simulink model "untitled"  (Simulink 7.3)
settings: Solver=ode45  StartTime=0.0  StopTime=10.0  RelTol=1e-3
settings Model: Creator=Sain  LastModifiedBy=Sain

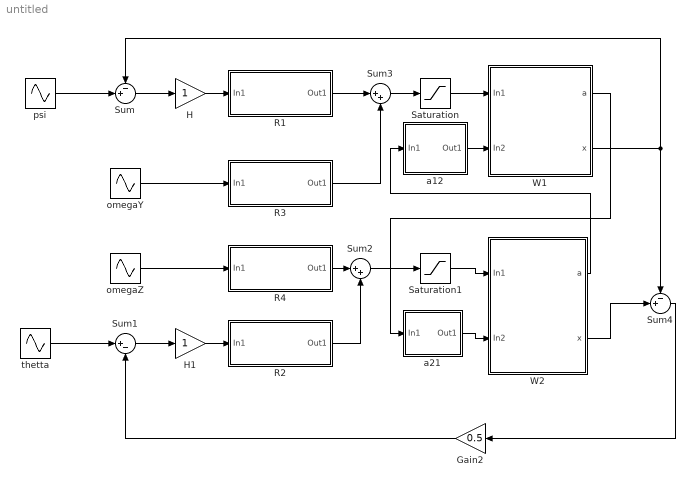
== system untitled ==
  Gain2 : Gain  Gain=0.5  ParameterDataType=fixdt(1, 16)  ParameterScaling=2^0  OutDataType=fixdt(1, 16)  OutScaling=2^0
  H : Gain  ParameterDataType=fixdt(1, 16)  ParameterScaling=2^0  OutDataType=fixdt(1, 16)  OutScaling=2^0
  H1 : Gain  ParameterDataType=fixdt(1, 16)  ParameterScaling=2^0  OutDataType=fixdt(1, 16)  OutScaling=2^0
  R1 : Subsystem
  R2 : Subsystem
  R3 : Subsystem
  R4 : Subsystem
  Saturation : Saturate  UpperLimit=27  LowerLimit=-27  OutDataType=fixdt(1, 16)  OutScaling=2^0
  Saturation1 : Saturate  UpperLimit=27  LowerLimit=-27  OutDataType=fixdt(1, 16)  OutScaling=2^0
  Sum : Sum  Inputs=-+|  OutDataType=fixdt(1, 16)  OutScaling=2^0
  Sum1 : Sum  Inputs=|+-  OutDataType=fixdt(1, 16)  OutScaling=2^0
  Sum2 : Sum  Inputs=|++  OutDataType=fixdt(1, 16)  OutScaling=2^0
  Sum3 : Sum  Inputs=|++  OutDataType=fixdt(1, 16)  OutScaling=2^0
  Sum4 : Sum  Inputs=-+|  OutDataType=fixdt(1, 16)  OutScaling=2^0
  W1 : Subsystem
  W2 : Subsystem
  a12 : Subsystem
  a21 : Subsystem
  omegaY : Sin  Amplitude=1  Bias=0  Frequency=1  Phase=0  Samples=10  SampleTime=0  Offset=0
  omegaZ : Sin  Amplitude=1  Bias=0  Frequency=1  Phase=0  Samples=10  SampleTime=0  Offset=0
  psi : Sin  Amplitude=1  Bias=0  Frequency=1  Phase=0  Samples=10  SampleTime=0  Offset=0
  thetta : Sin  Amplitude=1  Bias=0  Frequency=1  Phase=0  Samples=10  SampleTime=0  Offset=0
  wires:
  Sum/1 -> H/1
  Sum1/1 -> H1/1
  R2/1(Out1) -> Sum2/2
  R4/1(Out1) -> Sum2/1
  Sum2/1 -> Saturation1/1
  R1/1(Out1) -> Sum3/1
  Sum3/1 -> Saturation/1
  R3/1(Out1) -> Sum3/2
  H/1 -> R1/1(In1)
  Sum4/1 -> Gain2/1
  Gain2/1 -> Sum1/2
  Saturation1/1 -> W2/1(In1)
  a21/1(Out1) -> W2/2(In2)
  Saturation/1 -> W1/1(In1)
  a12/1(Out1) -> W1/2(In2)
  W1/2(x) -> Sum4/1, Sum/1
  W1/1(a) -> a21/1(In1)
  W2/1(a) -> a12/1(In1)
  W2/2(x) -> Sum4/2
  H1/1 -> R2/1(In1)
  omegaY/1 -> R3/1(In1)
  omegaZ/1 -> R4/1(In1)
  thetta/1 -> Sum1/1
  psi/1 -> Sum/2

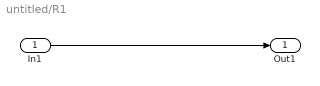
== system untitled/R1 ==
  In1 : Inport  OutDataType=fixdt(1, 16)  OutScaling=2^0
  Out1 : Outport  OutDataType=fixdt(1, 16)  OutScaling=2^0
  wires:
  In1/1 -> Out1/1

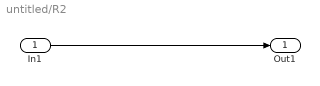
== system untitled/R2 ==
  In1 : Inport  OutDataType=fixdt(1, 16)  OutScaling=2^0
  Out1 : Outport  OutDataType=fixdt(1, 16)  OutScaling=2^0
  wires:
  In1/1 -> Out1/1

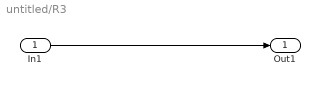
== system untitled/R3 ==
  In1 : Inport  OutDataType=fixdt(1, 16)  OutScaling=2^0
  Out1 : Outport  OutDataType=fixdt(1, 16)  OutScaling=2^0
  wires:
  In1/1 -> Out1/1

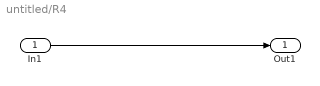
== system untitled/R4 ==
  In1 : Inport  OutDataType=fixdt(1, 16)  OutScaling=2^0
  Out1 : Outport  OutDataType=fixdt(1, 16)  OutScaling=2^0
  wires:
  In1/1 -> Out1/1

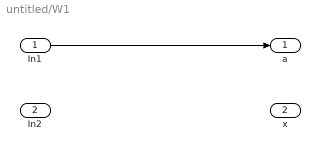
== system untitled/W1 ==
  In1 : Inport  OutDataType=fixdt(1, 16)  OutScaling=2^0
  In2 : Inport  Port=2  OutDataType=fixdt(1, 16)  OutScaling=2^0
  a : Outport  OutDataType=fixdt(1, 16)  OutScaling=2^0
  x : Outport  Port=2  OutDataType=fixdt(1, 16)  OutScaling=2^0
  wires:
  In1/1 -> a/1

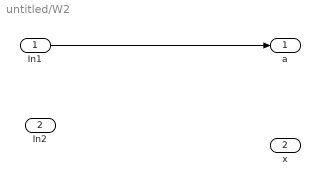
== system untitled/W2 ==
  In1 : Inport  OutDataType=fixdt(1, 16)  OutScaling=2^0
  In2 : Inport  Port=2  OutDataType=fixdt(1, 16)  OutScaling=2^0
  a : Outport  OutDataType=fixdt(1, 16)  OutScaling=2^0
  x : Outport  Port=2  OutDataType=fixdt(1, 16)  OutScaling=2^0
  wires:
  In1/1 -> a/1

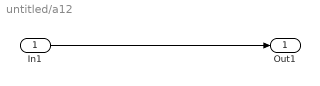
== system untitled/a12 ==
  In1 : Inport  OutDataType=fixdt(1, 16)  OutScaling=2^0
  Out1 : Outport  OutDataType=fixdt(1, 16)  OutScaling=2^0
  wires:
  In1/1 -> Out1/1

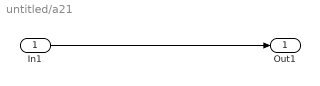
== system untitled/a21 ==
  In1 : Inport  OutDataType=fixdt(1, 16)  OutScaling=2^0
  Out1 : Outport  OutDataType=fixdt(1, 16)  OutScaling=2^0
  wires:
  In1/1 -> Out1/1
